simulink model "HOV"  (R2018b)
settings: Solver=VariableStepAuto  StartTime=0.0  StopTime=t_simul  RelTol=1e-3
values from neighbouring files (symbols this model uses):
  cc = 2*sqrt(m*ks)    [HalfVM.m]
undefined symbols (not defined in the file or in its folder): sigbuilder_block
libraries: fl_lib x28, nesl_utility x17, sdl_lib x2
settings Model: Creator=aliaramesh  LastModifiedBy=aliaramesh

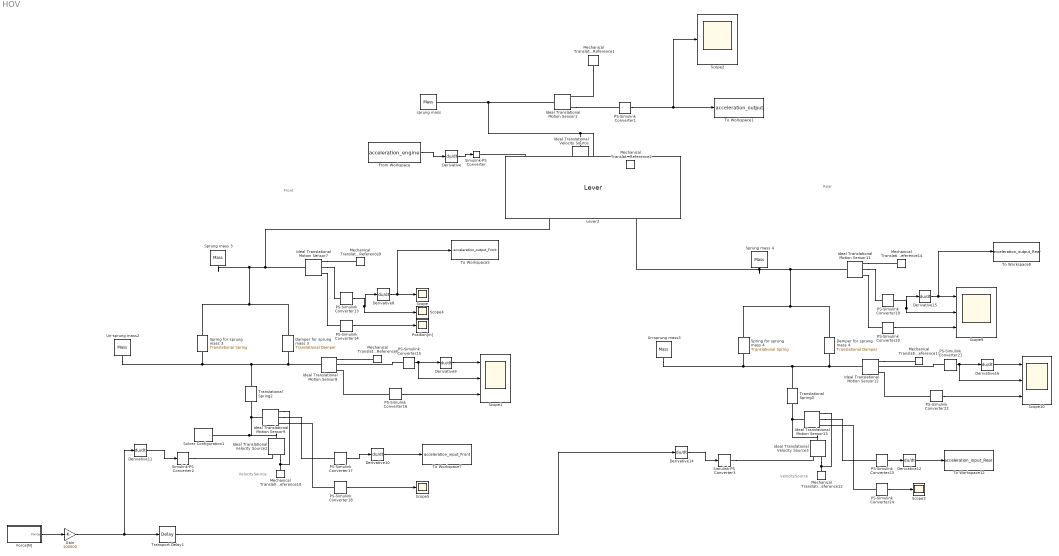
== system HOV ==
  note: Rear
  note: Front
  note: VelocitySource
  note: VelocitySource
  Damper for sprung mass 3 : sdl_lib/Couplings & Drives/Springs & Dampers/Translational Damper  D=cc N/(m/s)  enable_faults=0  b_fault=1e6 N/(m/s)  temporal_fault=0  fault_time=5 s  shock_fault=0  acceleration_limit=100 m/s^2  shock_limit=1  report_fault=1
      settings: SourceProductName=Simscape Driveline  SourceProductBaseCode=LD
  Damper for sprung mass 4 : sdl_lib/Couplings & Drives/Springs & Dampers/Translational Damper  D=cc N/(m/s)  enable_faults=0  b_fault=1e6 N/(m/s)  temporal_fault=0  fault_time=5 s  shock_fault=0  acceleration_limit=100 m/s^2  shock_limit=1  report_fault=1
      settings: SourceProductName=Simscape Driveline  SourceProductBaseCode=LD
  Derivative{,8..12,14..16} (9 alike) : Derivative
  "Force[N] " : Subsystem  Tag=STV Subsys  LoadFcn=sigbuilder_block('load');  StartFcn=sigbuilder_block('start');  StopFcn=sigbuilder_block('stop');  ClipboardFcn=sigbuilder_block('clipboard');  mask(Sigbuilder block){tuvar=[0:10]}
      mask help: Simulink:masks:SigbuilderBlock_MD
      mask init:
      | if ~strcmp(get_param(bdroot(gcbh),'SimulationStatus'),'stopped') tuvar = sigbuilder_block('maskInit'); end
      settings: CopyFcn=sigbuilder_block('copy');  DeleteFcn=sigbuilder_block('delete');  ModelCloseFcn=sigbuilder_block('modelClose');  PreSaveFcn=sigbuilder_block('preSave');  PauseFcn=sigbuilder_block('pause');  ContinueFcn=sigbuilder_block('continue');  NameChangeFcn=sigbuilder_block('namechange');  OpenFcn=sigbuilder_block('open',[437.6 199.2 550.4 400 ]);  CloseFcn=sigbuilder_block('close');
      mask Display: plot(0, 0, 100, 100,[2, 2, 32, 32, 2], [68, 8, 8, 68, 68],[32, 2], [38, 38], [32, 19, 2],[53, 60, 44], [32, 17, 17, 2],[16, 16, 31, 31]);txt = getActiveGroup(gcbh);text(2, 100, txt,'verticalAlignment', 'top');
  From Workspace : FromWorkspace  VariableName=acceleration_engine  SampleTime=0
  Gain : Gain  Gain=100000
  Ideal Translational Motion Sensor{1,7,9,11..13} (6 alike) : fl_lib/Mechanical/Mechanical Sensors/Ideal Translational Motion Sensor  offset=0 m
  Ideal Translational Motion Sensor8 : fl_lib/Mechanical/Mechanical Sensors/Ideal Translational Motion Sensor  offset=A_t m
  Ideal Translational Velocity Source : fl_lib/Mechanical/Mechanical Sources/Ideal Translational Velocity Source
  Ideal Translational Velocity Source2 : fl_lib/Mechanical/Mechanical Sources/Ideal Translational Velocity Source
  Ideal Translational Velocity Source3 : fl_lib/Mechanical/Mechanical Sources/Ideal Translational Velocity Source
  Lever2 : fl_lib/Mechanical/Mechanisms/Lever  arm_AC=0.1 m  arm_BC=0.1 m  f_A_specify=off  f_A_priority=None  f_A=0 N  f_A_nominal_specify=off  f_A_nominal_unit=N  f_A_nominal_value=1  f_B_specify=off  f_B_priority=None  f_B=0 N  f_B_nominal_specify=off  f_B_nominal_unit=N  f_B_nominal_value=1  f_C_specify=off  f_C_priority=None  f_C=0 N  f_C_nominal_specify=off  f_C_nominal_unit=N  f_C_nominal_value=1
      settings: SourceProductName=Simscape  SourceProductBaseCode=SS
  Mechanical Translational Reference{1..2,8..10,12..14} (8 alike) : fl_lib/Mechanical/Translational Elements/Mechanical Translational Reference
  PS-Simulink Converter{1,13,15..16,19..22} (8 alike) : nesl_utility/PS-Simulink Converter  PhysicalDomain=network_engine_domain  SubClassName=ps_output  LeftPortType=input  RightPortType=output  PseudoPeriodic=off  Frequencies=[]  Unit=1  AffineConversion=off
  PS-Simulink Converter14 : nesl_utility/PS-Simulink Converter  PhysicalDomain=network_engine_domain  SubClassName=ps_output  LeftPortType=input  RightPortType=output  PseudoPeriodic=off  Frequencies=[]  Unit=m  AffineConversion=off
  PS-Simulink Converter17 : nesl_utility/PS-Simulink Converter  PhysicalDomain=network_engine_domain  SubClassName=ps_output  LeftPortType=input  RightPortType=output  PseudoPeriodic=off  Frequencies=[]  Unit=m/s  AffineConversion=off
  PS-Simulink Converter18 : nesl_utility/PS-Simulink Converter  PhysicalDomain=network_engine_domain  SubClassName=ps_output  LeftPortType=input  RightPortType=output  PseudoPeriodic=off  Frequencies=[]  Unit=m  AffineConversion=off
  PS-Simulink Converter23 : nesl_utility/PS-Simulink Converter  PhysicalDomain=network_engine_domain  SubClassName=ps_output  LeftPortType=input  RightPortType=output  PseudoPeriodic=off  Frequencies=[]  Unit=m/s  AffineConversion=off
  PS-Simulink Converter24 : nesl_utility/PS-Simulink Converter  PhysicalDomain=network_engine_domain  SubClassName=ps_output  LeftPortType=input  RightPortType=output  PseudoPeriodic=off  Frequencies=[]  Unit=m  AffineConversion=off
  Position[m] : Scope
  Scope{,2..5} (5 alike) : Scope
  Scope1 : Scope  NumInputPorts=3
  Scope10 : Scope  NumInputPorts=3
  Scope9 : Scope  NumInputPorts=3
  Simulink-PS Converter : nesl_utility/Simulink-PS Converter  PhysicalDomain=network_engine_domain  SubClassName=ps_input  LeftPortType=input  RightPortType=output  PseudoPeriodic=off  Frequencies=[]  NoiseDistribution=none  NoiseParameters=[]  Unit=1  AffineConversion=off  FilteringAndDerivatives=provide  SimscapeFilterOrder=1  InputFilterTimeConstant=0.001  UdotUserProvided=0
  Simulink-PS Converter2 : nesl_utility/Simulink-PS Converter  PhysicalDomain=network_engine_domain  SubClassName=ps_input  LeftPortType=input  RightPortType=output  PseudoPeriodic=off  Frequencies=[]  NoiseDistribution=none  NoiseParameters=[]  Unit=m/s  AffineConversion=off  FilteringAndDerivatives=provide  SimscapeFilterOrder=1  InputFilterTimeConstant=0.001  UdotUserProvided=0
  Simulink-PS Converter3 : nesl_utility/Simulink-PS Converter  PhysicalDomain=network_engine_domain  SubClassName=ps_input  LeftPortType=input  RightPortType=output  PseudoPeriodic=off  Frequencies=[]  NoiseDistribution=none  NoiseParameters=[]  Unit=m/s  AffineConversion=off  FilteringAndDerivatives=provide  SimscapeFilterOrder=1  InputFilterTimeConstant=0.001  UdotUserProvided=0
  Solver Configuration1 : nesl_utility/Solver Configuration  PhysicalDomain=network_engine_domain  SubClassName=solver  LeftPortType=input  RightPortType=generic  Tones=[]  Harmonics=[]  SimulateNoise=off  Profile=off  UseLocalSampling=off  EnableSwitchedLinearOptims=on  FrequencyDomain=off  UseCCode=off  RelTol=0.001  AbsTol=1e-06  MinStep=1e-09  ToWorkspace=off  RevertToSquareIcSolve=off  NumHomotopyIterations=100  PhasorMode=off  PhasorModeNumHarmonics=1  DoDC=off  ResidualTolerance=1e-09  UseLocalSolver=off  LocalSolverChoice=NE_BACKWARD_EULER_ADVANCER  LocalSolverSampleTime=0.001  DoFixedCost=off  MaxNonlinIter=3  MaxModeIter=2  LinearAlgebra=Sparse  EquationFormulation=NE_TIME_EF  DelaysMemoryBudget=1024  AutomaticFiltering=on  FilteringTimeConstant=0.001  PartitionStorageMethod=AS_NEEDED  PartitionMemoryBudget=1024
  Spring for sprung mass 3 : fl_lib/Mechanical/Translational Elements/Translational Spring  spr_rate=ks N/m  v_specify=off  v_priority=None  v=0 m/s  v_nominal_specify=off  v_nominal_unit=m/s  v_nominal_value=1  f_specify=off  f_priority=None  f=0 N  f_nominal_specify=off  f_nominal_unit=N  f_nominal_value=1  x_specify=off  x_priority=High  x=0 m  x_nominal_specify=off  x_nominal_unit=m  x_nominal_value=1
  Spring for sprung mass 4 : fl_lib/Mechanical/Translational Elements/Translational Spring  spr_rate=ks N/m  v_specify=off  v_priority=None  v=0 m/s  v_nominal_specify=off  v_nominal_unit=m/s  v_nominal_value=1  f_specify=off  f_priority=None  f=0 N  f_nominal_specify=off  f_nominal_unit=N  f_nominal_value=1  x_specify=off  x_priority=High  x=0 m  x_nominal_specify=off  x_nominal_unit=m  x_nominal_value=1
  Sprung mass 3 : fl_lib/Mechanical/Translational Elements/Mass  mass=mc kg  v_specify=off  v_priority=High  v=0 m/s  v_nominal_specify=off  v_nominal_unit=m/s  v_nominal_value=1  f_specify=off  f_priority=None  f=0 N  f_nominal_specify=off  f_nominal_unit=N  f_nominal_value=1
  Sprung mass 4 : fl_lib/Mechanical/Translational Elements/Mass  mass=mc kg  v_specify=off  v_priority=High  v=0 m/s  v_nominal_specify=off  v_nominal_unit=m/s  v_nominal_value=1  f_specify=off  f_priority=None  f=0 N  f_nominal_specify=off  f_nominal_unit=N  f_nominal_value=1
  To Workspace1 : ToWorkspace  VariableName=acceleration_output  SampleTime=-1
  To Workspace12 : ToWorkspace  VariableName=acceleration_input_Rear  SampleTime=-1
  To Workspace5 : ToWorkspace  VariableName=acceleration_output_Front  SampleTime=-1
  To Workspace7 : ToWorkspace  VariableName=acceleration_input_Front  SampleTime=-1
  To Workspace8 : ToWorkspace  VariableName=acceleration_output_Rear  SampleTime=-1
  Translational Spring2 : fl_lib/Mechanical/Translational Elements/Translational Spring  spr_rate=kw N/m  v_specify=off  v_priority=None  v=0 m/s  v_nominal_specify=off  v_nominal_unit=m/s  v_nominal_value=1  f_specify=off  f_priority=None  f=0 N  f_nominal_specify=off  f_nominal_unit=N  f_nominal_value=1  x_specify=off  x_priority=High  x=0 m  x_nominal_specify=off  x_nominal_unit=m  x_nominal_value=1
  Translational Spring3 : fl_lib/Mechanical/Translational Elements/Translational Spring  spr_rate=kw N/m  v_specify=off  v_priority=None  v=0 m/s  v_nominal_specify=off  v_nominal_unit=m/s  v_nominal_value=1  f_specify=off  f_priority=None  f=0 N  f_nominal_specify=off  f_nominal_unit=N  f_nominal_value=1  x_specify=off  x_priority=High  x=0 m  x_nominal_specify=off  x_nominal_unit=m  x_nominal_value=1
  Transport Delay1 : TransportDelay
  Un-sprung mass2 : fl_lib/Mechanical/Translational Elements/Mass  mass=mw kg  v_specify=off  v_priority=High  v=0 m/s  v_nominal_specify=off  v_nominal_unit=m/s  v_nominal_value=1  f_specify=off  f_priority=None  f=0 N  f_nominal_specify=off  f_nominal_unit=N  f_nominal_value=1
  Un-sprung mass3 : fl_lib/Mechanical/Translational Elements/Mass  mass=mw kg  v_specify=off  v_priority=High  v=0 m/s  v_nominal_specify=off  v_nominal_unit=m/s  v_nominal_value=1  f_specify=off  f_priority=None  f=0 N  f_nominal_specify=off  f_nominal_unit=N  f_nominal_value=1
  "sprung mass " : fl_lib/Mechanical/Translational Elements/Mass  mass=500 kg  v_specify=off  v_priority=High  v=0 m/s  v_nominal_specify=off  v_nominal_unit=m/s  v_nominal_value=1  f_specify=off  f_priority=None  f=0 N  f_nominal_specify=off  f_nominal_unit=N  f_nominal_value=1
  wires:
  Derivative10/1 -> To Workspace7/1
  Derivative9/1 -> Scope1/1
  PS-Simulink Converter17/1 -> Derivative10/1
  Gain/1 -> Transport Delay1/1, Derivative11/1
  PS-Simulink Converter14/1 -> Position[m]/1
  PS-Simulink Converter15/1 -> Scope1/2, Derivative9/1
  Derivative11/1 -> Simulink-PS Converter2/1
  PS-Simulink Converter13/1 -> Scope4/1, Derivative8/1
  PS-Simulink Converter18/1 -> Scope5/1
  Derivative8/1 -> Scope/1, To Workspace5/1
  PS-Simulink Converter16/1 -> Scope1/3
  PS-Simulink Converter22/1 -> Scope10/3
  Derivative15/1 -> Scope9/1, To Workspace8/1
  PS-Simulink Converter24/1 -> Scope3/1
  PS-Simulink Converter19/1 -> Derivative15/1, Scope9/2
  Derivative14/1 -> Simulink-PS Converter3/1
  PS-Simulink Converter21/1 -> Derivative16/1, Scope10/2
  PS-Simulink Converter20/1 -> Scope9/3
  PS-Simulink Converter23/1 -> Derivative12/1
  Derivative16/1 -> Scope10/1
  Derivative12/1 -> To Workspace12/1
  PS-Simulink Converter1/1 -> Scope2/1, To Workspace1/1
  "Force[N] "/1(Force) -> Gain/1
  Transport Delay1/1 -> Derivative14/1
  Derivative/1 -> Simulink-PS Converter/1
  From Workspace/1 -> Derivative/1
  connections:
  Mechanical Translational Reference10/LConn1 -- Ideal Translational Velocity Source2/RConn2 -- Ideal Translational Motion Sensor9/RConn1
  Translational Spring2/RConn1 -- Un-sprung mass2/LConn1 -- Spring for sprung mass 3/RConn1 -- Ideal Translational Motion Sensor8/LConn1 -- Damper for sprung mass 3/RConn1
  Spring for sprung mass 3/LConn1 -- Damper for sprung mass 3/LConn1 -- Ideal Translational Motion Sensor7/LConn1 -- Lever2/LConn1 -- Sprung mass 3/LConn1
  Ideal Translational Velocity Source2/LConn1 -- Solver Configuration1/RConn1 -- Ideal Translational Motion Sensor9/LConn1 -- Translational Spring2/LConn1
  Ideal Translational Motion Sensor7/RConn2 -- PS-Simulink Converter13/LConn1
  Ideal Translational Motion Sensor9/RConn2 -- PS-Simulink Converter17/LConn1
  PS-Simulink Converter16/LConn1 -- Ideal Translational Motion Sensor8/RConn3
  PS-Simulink Converter18/LConn1 -- Ideal Translational Motion Sensor9/RConn3
  PS-Simulink Converter15/LConn1 -- Ideal Translational Motion Sensor8/RConn2
  Simulink-PS Converter2/RConn1 -- Ideal Translational Velocity Source2/RConn1
  Ideal Translational Motion Sensor7/RConn3 -- PS-Simulink Converter14/LConn1
  Ideal Translational Motion Sensor8/RConn1 -- Mechanical Translational Reference8/LConn1
  Ideal Translational Motion Sensor7/RConn1 -- Mechanical Translational Reference9/LConn1
  Ideal Translational Velocity Source3/RConn2 -- Mechanical Translational Reference12/LConn1 -- Ideal Translational Motion Sensor13/RConn1
  Ideal Translational Motion Sensor12/LConn1 -- Translational Spring3/RConn1 -- Spring for sprung mass 4/RConn1 -- Un-sprung mass3/LConn1 -- Damper for sprung mass 4/RConn1
  Damper for sprung mass 4/LConn1 -- Ideal Translational Motion Sensor11/LConn1 -- Sprung mass 4/LConn1 -- Lever2/LConn2 -- Spring for sprung mass 4/LConn1
  Ideal Translational Motion Sensor13/LConn1 -- Ideal Translational Velocity Source3/LConn1 -- Translational Spring3/LConn1
  Ideal Translational Motion Sensor11/RConn1 -- Mechanical Translational Reference14/LConn1
  PS-Simulink Converter22/LConn1 -- Ideal Translational Motion Sensor12/RConn3
  Ideal Translational Motion Sensor11/RConn2 -- PS-Simulink Converter19/LConn1
  Ideal Translational Motion Sensor13/RConn2 -- PS-Simulink Converter23/LConn1
  PS-Simulink Converter24/LConn1 -- Ideal Translational Motion Sensor13/RConn3
  PS-Simulink Converter21/LConn1 -- Ideal Translational Motion Sensor12/RConn2
  Simulink-PS Converter3/RConn1 -- Ideal Translational Velocity Source3/RConn1
  Ideal Translational Motion Sensor11/RConn3 -- PS-Simulink Converter20/LConn1
  Ideal Translational Motion Sensor12/RConn1 -- Mechanical Translational Reference13/LConn1
  Ideal Translational Motion Sensor1/RConn3 -- PS-Simulink Converter1/LConn1
  Mechanical Translational Reference1/LConn1 -- Ideal Translational Motion Sensor1/RConn1
  Ideal Translational Motion Sensor1/LConn1 -- Ideal Translational Velocity Source/LConn1 -- Lever2/RConn1 -- "sprung mass "/LConn1
  Ideal Translational Velocity Source/RConn2 -- Mechanical Translational Reference2/LConn1
  Ideal Translational Velocity Source/RConn1 -- Simulink-PS Converter/RConn1

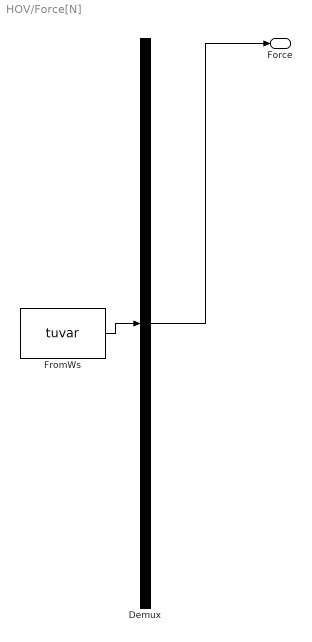
== system HOV/Force[N]  ==
  Demux : Demux  Tag=STV Demux  Outputs=1
  FromWs : FromWorkspace  Tag=STV FromWs  VariableName=tuvar  SampleTime=0
      SigBuilderData=|
      | common.afterFinalStr = 'Extrapolate'
      | common.sampleTime = 0
      | dataSet.timeRange = [0 10]
      | dataSet.name = 'Group 1'
      | sbobj.Groups.Name = 'Group 1'
      | sbobj.Groups.Signals.Name = 'Force'
      | sbobj.Groups.Signals.XData = [0 3.05 3.05 6 6 10]
      | sbobj.Groups.Signals.YData = [0 0 1 1.005 0 0]
  Force : Outport  Tag=STV Outport
  wires:
  Demux/1 -> Force/1
  FromWs/1 -> Demux/1
